simulink model "w1p2"  (R2020b)
settings: Solver=VariableStepAuto  StartTime=0.0  StopTime=10.0  RelTol=1e-3
undefined symbols (not defined in the file): b, K1, K2, M1, M2
settings Model: Creator=Dell  LastModifiedBy=Dell

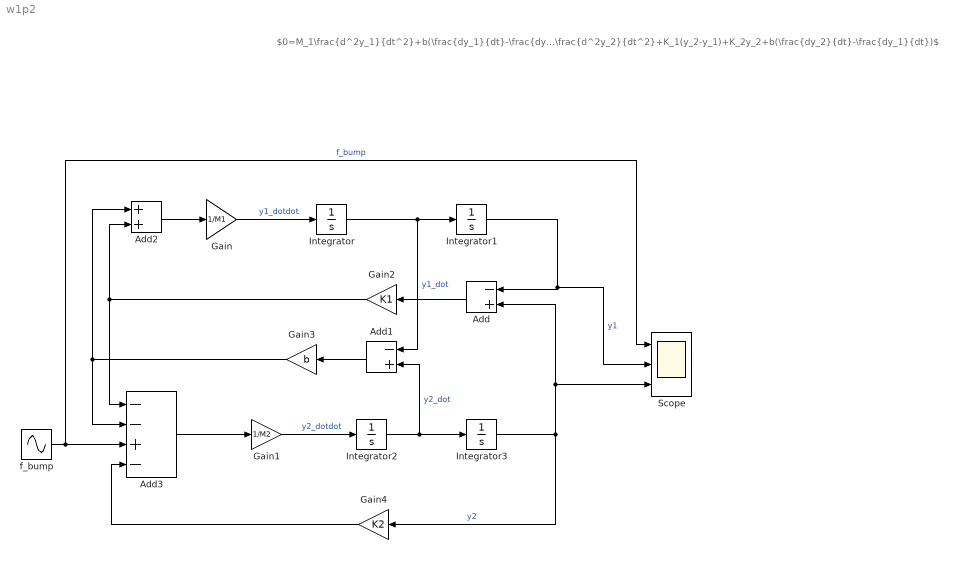
== system w1p2 ==
  note: $0=M_1\frac{d^2y_1}{dt^2}+b(\frac{dy_1}{dt}-\frac{dy_2}{dt})+K_1(y_1-y_2)\\f_{bump}=M_2\frac{d^2y_2}{dt^2}+K_1(y_2-y_1)+K_2y_2+b(\frac{dy_2}{dt}-\frac{dy_1}{dt})$
  Add : Sum  Inputs=-+
  Add1 : Sum  Inputs=-+
  Add2 : Sum
  Add3 : Sum  Inputs=--+-
  Gain : Gain  Gain=1/M1
  Gain1 : Gain  Gain=1/M2
  Gain2 : Gain  Gain=K1
  Gain3 : Gain  Gain=b
  Gain4 : Gain  Gain=K2
  Integrator{,1..3} (4 alike) : Integrator
  Scope : Scope  NumInputPorts=3
  f_bump : Sin  SampleTime=0
  wires:
  Gain/1 -> Integrator/1  "y1_dotdot"
  Integrator/1 -> Add1/1, Integrator1/1  "y1_dot"
  Integrator2/1 -> Add1/2, Integrator3/1  "y2_dot"
  Gain1/1 -> Integrator2/1  "y2_dotdot"
  Integrator1/1 -> Scope/2, Add/1  "y1"
  Integrator3/1 -> Add/2, Scope/3, Gain4/1  "y2"
  Add/1 -> Gain2/1
  Gain2/1 -> Add2/2, Add3/1
  Add1/1 -> Gain3/1
  Gain3/1 -> Add3/2, Add2/1
  Add3/1 -> Gain1/1
  Add2/1 -> Gain/1
  Gain4/1 -> Add3/4
  f_bump/1 -> Scope/1, Add3/3  "f_bump"
